simulink model "sys"  (R2024a)
settings: Solver=VariableStepAuto  StartTime=0.0  StopTime=2e-3  RelTol=1e-3
libraries: dspsigops x11, commdigbbndpm3 x1, commrandsrc3 x1, simulink x1
(part 1 of 2)
settings Model: Creator=abc  LastModifiedBy=abc

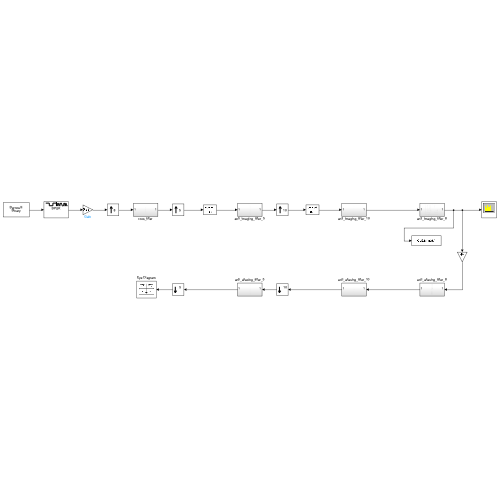
[thumbnail: Simulink's stored preview of the top-level diagram]
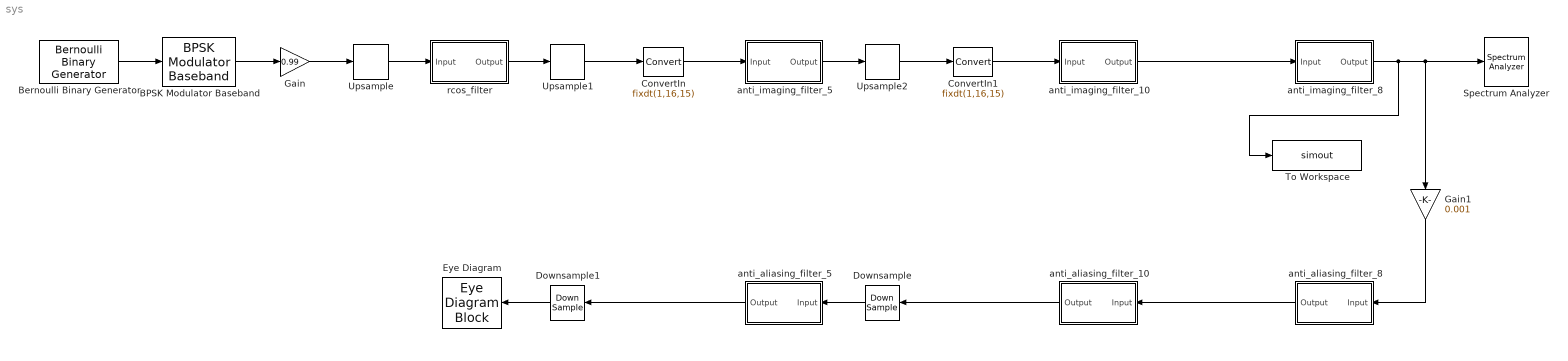
== system sys ==
  BPSK Modulator Baseband : commdigbbndpm3/BPSK Modulator Baseband  Ph=0  outDtype=double  outWordLen=16  outUDDataType=sfix(16)  outFracLenMode=Best precision  outFracLen=15  outDataTypeStr=double  outLastDataTypeStr=double
  Bernoulli Binary Generator : commrandsrc3/Bernoulli Binary Generator  ProbabilityOfZero=0.5  SeedSource=Auto  Seed=0  SampleTime=1/(450e3)  SamplesPerFrame=1  OutputDataType=double  SimulateUsing=Interpreted execution
  ConvertIn : DataTypeConversion  OutDataTypeStr=fixdt(1,16,15)  ConvertRealWorld=Stored Integer (SI)  RndMeth=Nearest
  ConvertIn1 : DataTypeConversion  OutDataTypeStr=fixdt(1,16,15)  ConvertRealWorld=Stored Integer (SI)  RndMeth=Nearest
  Downsample : DownSample  N=10  RateOptions=Allow multirate processing  AllowArbitraryFixedInput=on
  Downsample1 : DownSample  N=5  RateOptions=Allow multirate processing  AllowArbitraryFixedInput=on
  Eye Diagram : EyeDiagramBlock  WindowPosition=[302.000000,120.000000,800.000000,500.000000,]  ScopeFrameLocation=window  YLimits=[-2.8631442273035645,3.1513396510854363]  PlotImaginaryAxes=off
  Gain : Gain  Gain=0.99
  Gain1 : Gain  Gain=0.001
  Spectrum Analyzer : SpectrumAnalyzer  WindowPosition=[48.000000,117.000000,800.000000,500.000000,]  ScopeFrameLocation=window  SampleRateSource=Property  SampleRate=1  Span=3600000.0000000005  StartFrequency=-1800000.0000000002  StopFrequency=1800000.0000000002  YLimits=[-122.72965629,37.88911859]  ExpandToolstrip=on
  To Workspace : ToWorkspace  VariableName=simout  SampleTime=-1
      settings: Save2DSignal=2-D array (concatenate along first dimension)
  Upsample : dspsigops/Upsample  FactorSource=Dialog parameter  N=8  Nmax=16  phase=0  InputProcessing=Columns as channels (frame based)  RateOptions=Allow multirate processing  ic=0  mode=Unused parameter value
  Upsample1 : dspsigops/Upsample  FactorSource=Dialog parameter  N=5  Nmax=16  phase=0  InputProcessing=Columns as channels (frame based)  RateOptions=Allow multirate processing  ic=0  mode=Unused parameter value
  Upsample2 : dspsigops/Upsample  FactorSource=Dialog parameter  N=10  Nmax=16  phase=0  InputProcessing=Columns as channels (frame based)  RateOptions=Allow multirate processing  ic=0  mode=Unused parameter value
  anti_aliasing_filter_10 : Subsystem  Tag=FilterWizardSubSystem
      settings: ErrorFcn=dspFilterRealizedInBasicElemsAlgLoopErrFcnCallback
  anti_aliasing_filter_5 : Subsystem  Tag=FilterWizardSubSystem
      settings: ErrorFcn=dspFilterRealizedInBasicElemsAlgLoopErrFcnCallback
  anti_aliasing_filter_8 : Subsystem  Tag=FilterWizardSubSystem
      settings: ErrorFcn=dspFilterRealizedInBasicElemsAlgLoopErrFcnCallback
  anti_imaging_filter_10 : Subsystem  Tag=FilterWizardSubSystem
      settings: ErrorFcn=dspFilterRealizedInBasicElemsAlgLoopErrFcnCallback
  anti_imaging_filter_5 : Subsystem  Tag=FilterWizardSubSystem
      settings: ErrorFcn=dspFilterRealizedInBasicElemsAlgLoopErrFcnCallback
  anti_imaging_filter_8 : Subsystem  Tag=FilterWizardSubSystem
      settings: ErrorFcn=dspFilterRealizedInBasicElemsAlgLoopErrFcnCallback
  rcos_filter : Subsystem  Tag=FilterWizardSubSystem
      settings: ErrorFcn=dspFilterRealizedInBasicElemsAlgLoopErrFcnCallback
  wires:
  Bernoulli Binary Generator/1 -> BPSK Modulator Baseband/1
  BPSK Modulator Baseband/1 -> Gain/1
  Upsample/1 -> rcos_filter/1(Input)
  rcos_filter/1(Output) -> Upsample1/1
  anti_imaging_filter_5/1(Output) -> Upsample2/1
  Downsample/1 -> anti_aliasing_filter_5/1(Input)
  anti_aliasing_filter_5/1(Output) -> Downsample1/1
  anti_aliasing_filter_8/1(Output) -> anti_aliasing_filter_10/1(Input)
  anti_aliasing_filter_10/1(Output) -> Downsample/1
  Gain/1 -> Upsample/1
  Upsample1/1 -> ConvertIn/1
  Upsample2/1 -> ConvertIn1/1
  anti_imaging_filter_8/1(Output) -> To Workspace/1, Gain1/1, Spectrum Analyzer/1
  ConvertIn/1 -> anti_imaging_filter_5/1(Input)
  ConvertIn1/1 -> anti_imaging_filter_10/1(Input)
  Downsample1/1 -> Eye Diagram/1
  anti_imaging_filter_10/1(Output) -> anti_imaging_filter_8/1(Input)
  Gain1/1 -> anti_aliasing_filter_8/1(Input)

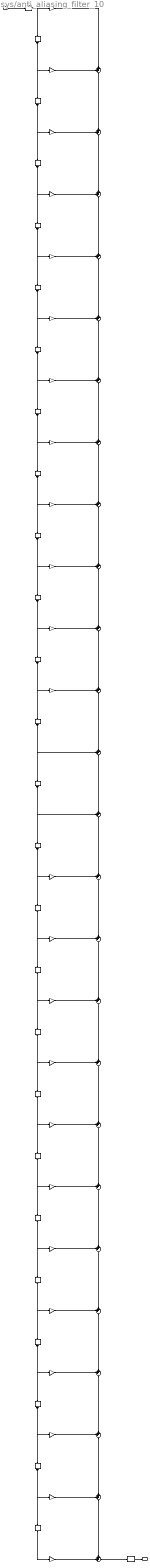
== system sys/anti_aliasing_filter_10 ==
  Input : Inport
  BodyDelay{2..26} (25 alike) : Delay  DelayLength=1  InitialCondition=0
  BodyLSum{2..26} (25 alike) : Sum  Inputs=++|  OutDataTypeStr=fixdt(1,35,30)  AccumDataTypeStr=fixdt(1,35,30)  RndMeth=Convergent
  ConvertIn : DataTypeConversion  OutDataTypeStr=fixdt(1,16,15)  RndMeth=Nearest
  ConvertOut : DataTypeConversion  OutDataTypeStr=fixdt(1,15,14)  RndMeth=Convergent  SaturateOnIntegerOverflow=off
  b(1) : Gain  Gain=0.0156626064233622506  ParamDataTypeStr=fixdt(1,16,15)  OutDataTypeStr=fixdt(1,31,30)  RndMeth=Convergent
  b(10) : Gain  Gain=0.784930628612014125  ParamDataTypeStr=fixdt(1,16,15)  OutDataTypeStr=fixdt(1,31,30)  RndMeth=Convergent
  b(11) : Gain  Gain=0.886772527356170293  ParamDataTypeStr=fixdt(1,16,15)  OutDataTypeStr=fixdt(1,31,30)  RndMeth=Convergent
  b(12) : Gain  Gain=0.960925295623340392  ParamDataTypeStr=fixdt(1,16,15)  OutDataTypeStr=fixdt(1,31,30)  RndMeth=Convergent
  b(15) : Gain  Gain=0.960925295623340392  ParamDataTypeStr=fixdt(1,16,15)  OutDataTypeStr=fixdt(1,31,30)  RndMeth=Convergent
  b(16) : Gain  Gain=0.886772527356170293  ParamDataTypeStr=fixdt(1,16,15)  OutDataTypeStr=fixdt(1,31,30)  RndMeth=Convergent
  b(17) : Gain  Gain=0.784930628612014125  ParamDataTypeStr=fixdt(1,16,15)  OutDataTypeStr=fixdt(1,31,30)  RndMeth=Convergent
  b(18) : Gain  Gain=0.665103266921935554  ParamDataTypeStr=fixdt(1,16,15)  OutDataTypeStr=fixdt(1,31,30)  RndMeth=Convergent
  b(19) : Gain  Gain=0.537919174813016099  ParamDataTypeStr=fixdt(1,16,15)  OutDataTypeStr=fixdt(1,31,30)  RndMeth=Convergent
  b(2) : Gain  Gain=0.0362761924333834043  ParamDataTypeStr=fixdt(1,16,15)  OutDataTypeStr=fixdt(1,31,30)  RndMeth=Convergent
  b(20) : Gain  Gain=0.413536705569194474  ParamDataTypeStr=fixdt(1,16,15)  OutDataTypeStr=fixdt(1,31,30)  RndMeth=Convergent
  b(21) : Gain  Gain=0.30040563304203749  ParamDataTypeStr=fixdt(1,16,15)  OutDataTypeStr=fixdt(1,31,30)  RndMeth=Convergent
  b(22) : Gain  Gain=0.204429372845306323  ParamDataTypeStr=fixdt(1,16,15)  OutDataTypeStr=fixdt(1,31,30)  RndMeth=Convergent
  b(23) : Gain  Gain=0.128628263180761093  ParamDataTypeStr=fixdt(1,16,15)  OutDataTypeStr=fixdt(1,31,30)  RndMeth=Convergent
  b(24) : Gain  Gain=0.0732387285445653402  ParamDataTypeStr=fixdt(1,16,15)  OutDataTypeStr=fixdt(1,31,30)  RndMeth=Convergent
  b(25) : Gain  Gain=0.0362761924333834043  ParamDataTypeStr=fixdt(1,16,15)  OutDataTypeStr=fixdt(1,31,30)  RndMeth=Convergent
  b(26) : Gain  Gain=0.0156626064233622506  ParamDataTypeStr=fixdt(1,16,15)  OutDataTypeStr=fixdt(1,31,30)  RndMeth=Convergent
  b(3) : Gain  Gain=0.0732387285445653402  ParamDataTypeStr=fixdt(1,16,15)  OutDataTypeStr=fixdt(1,31,30)  RndMeth=Convergent
  b(4) : Gain  Gain=0.128628263180761093  ParamDataTypeStr=fixdt(1,16,15)  OutDataTypeStr=fixdt(1,31,30)  RndMeth=Convergent
  b(5) : Gain  Gain=0.204429372845306323  ParamDataTypeStr=fixdt(1,16,15)  OutDataTypeStr=fixdt(1,31,30)  RndMeth=Convergent
  b(6) : Gain  Gain=0.30040563304203749  ParamDataTypeStr=fixdt(1,16,15)  OutDataTypeStr=fixdt(1,31,30)  RndMeth=Convergent
  b(7) : Gain  Gain=0.413536705569194474  ParamDataTypeStr=fixdt(1,16,15)  OutDataTypeStr=fixdt(1,31,30)  RndMeth=Convergent
  b(8) : Gain  Gain=0.537919174813016099  ParamDataTypeStr=fixdt(1,16,15)  OutDataTypeStr=fixdt(1,31,30)  RndMeth=Convergent
  b(9) : Gain  Gain=0.665103266921935554  ParamDataTypeStr=fixdt(1,16,15)  OutDataTypeStr=fixdt(1,31,30)  RndMeth=Convergent
  Output : Outport
  wires:
  Input/1 -> ConvertIn/1
  b(1)/1 -> BodyLSum2/2
  ConvertIn/1 -> b(1)/1, BodyDelay2/1
  BodyDelay2/1 -> b(2)/1, BodyDelay3/1
  b(2)/1 -> BodyLSum2/1
  BodyLSum2/1 -> BodyLSum3/2
  BodyDelay3/1 -> b(3)/1, BodyDelay4/1
  b(3)/1 -> BodyLSum3/1
  BodyLSum3/1 -> BodyLSum4/2
  BodyDelay4/1 -> b(4)/1, BodyDelay5/1
  b(4)/1 -> BodyLSum4/1
  BodyLSum4/1 -> BodyLSum5/2
  BodyDelay5/1 -> b(5)/1, BodyDelay6/1
  b(5)/1 -> BodyLSum5/1
  BodyLSum5/1 -> BodyLSum6/2
  BodyDelay6/1 -> b(6)/1, BodyDelay7/1
  b(6)/1 -> BodyLSum6/1
  BodyLSum6/1 -> BodyLSum7/2
  BodyDelay7/1 -> b(7)/1, BodyDelay8/1
  b(7)/1 -> BodyLSum7/1
  BodyLSum7/1 -> BodyLSum8/2
  BodyDelay8/1 -> b(8)/1, BodyDelay9/1
  b(8)/1 -> BodyLSum8/1
  BodyLSum8/1 -> BodyLSum9/2
  BodyDelay9/1 -> b(9)/1, BodyDelay10/1
  b(9)/1 -> BodyLSum9/1
  BodyLSum9/1 -> BodyLSum10/2
  BodyDelay10/1 -> b(10)/1, BodyDelay11/1
  b(10)/1 -> BodyLSum10/1
  BodyLSum10/1 -> BodyLSum11/2
  BodyDelay11/1 -> b(11)/1, BodyDelay12/1
  b(11)/1 -> BodyLSum11/1
  BodyLSum11/1 -> BodyLSum12/2
  BodyDelay12/1 -> b(12)/1, BodyDelay13/1
  b(12)/1 -> BodyLSum12/1
  BodyLSum12/1 -> BodyLSum13/2
  BodyDelay13/1 -> BodyLSum13/1, BodyDelay14/1
  BodyLSum13/1 -> BodyLSum14/2
  BodyDelay14/1 -> BodyLSum14/1, BodyDelay15/1
  BodyLSum14/1 -> BodyLSum15/2
  BodyDelay15/1 -> b(15)/1, BodyDelay16/1
  b(15)/1 -> BodyLSum15/1
  BodyLSum15/1 -> BodyLSum16/2
  BodyDelay16/1 -> b(16)/1, BodyDelay17/1
  b(16)/1 -> BodyLSum16/1
  BodyLSum16/1 -> BodyLSum17/2
  BodyDelay17/1 -> b(17)/1, BodyDelay18/1
  b(17)/1 -> BodyLSum17/1
  BodyLSum17/1 -> BodyLSum18/2
  BodyDelay18/1 -> b(18)/1, BodyDelay19/1
  b(18)/1 -> BodyLSum18/1
  BodyLSum18/1 -> BodyLSum19/2
  BodyDelay19/1 -> b(19)/1, BodyDelay20/1
  b(19)/1 -> BodyLSum19/1
  BodyLSum19/1 -> BodyLSum20/2
  BodyDelay20/1 -> b(20)/1, BodyDelay21/1
  b(20)/1 -> BodyLSum20/1
  BodyLSum20/1 -> BodyLSum21/2
  BodyDelay21/1 -> b(21)/1, BodyDelay22/1
  b(21)/1 -> BodyLSum21/1
  BodyLSum21/1 -> BodyLSum22/2
  BodyDelay22/1 -> b(22)/1, BodyDelay23/1
  b(22)/1 -> BodyLSum22/1
  BodyLSum22/1 -> BodyLSum23/2
  BodyDelay23/1 -> b(23)/1, BodyDelay24/1
  b(23)/1 -> BodyLSum23/1
  BodyLSum23/1 -> BodyLSum24/2
  BodyDelay24/1 -> b(24)/1, BodyDelay25/1
  b(24)/1 -> BodyLSum24/1
  BodyLSum24/1 -> BodyLSum25/2
  BodyDelay25/1 -> b(25)/1, BodyDelay26/1
  b(25)/1 -> BodyLSum25/1
  BodyLSum25/1 -> BodyLSum26/1
  BodyDelay26/1 -> b(26)/1
  b(26)/1 -> BodyLSum26/2
  BodyLSum26/1 -> ConvertOut/1
  ConvertOut/1 -> Output/1

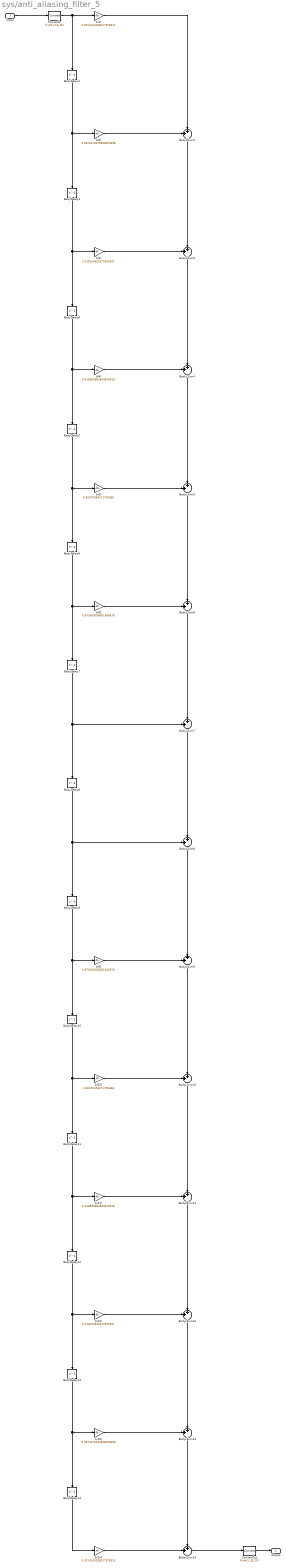
== system sys/anti_aliasing_filter_5 ==
  Input : Inport
  BodyDelay{2..14} (13 alike) : Delay  DelayLength=1  InitialCondition=0
  BodyLSum{2..14} (13 alike) : Sum  Inputs=++|  OutDataTypeStr=fixdt(1,33,29)  AccumDataTypeStr=fixdt(1,33,29)  RndMeth=Convergent
  ConvertIn : DataTypeConversion  OutDataTypeStr=fixdt(1,16,15)  RndMeth=Nearest
  ConvertOut : DataTypeConversion  OutDataTypeStr=fixdt(1,33,29)  RndMeth=Convergent  SaturateOnIntegerOverflow=off
  b(1) : Gain  Gain=0.0224233208217978312  ParamDataTypeStr=fixdt(1,16,14)  OutDataTypeStr=fixdt(1,31,29)  RndMeth=Convergent
  b(10) : Gain  Gain=0.65370494271794366  ParamDataTypeStr=fixdt(1,16,14)  OutDataTypeStr=fixdt(1,31,29)  RndMeth=Convergent
  b(11) : Gain  Gain=0.416892883843040518  ParamDataTypeStr=fixdt(1,16,14)  OutDataTypeStr=fixdt(1,31,29)  RndMeth=Convergent
  b(12) : Gain  Gain=0.218154593372955397  ParamDataTypeStr=fixdt(1,16,14)  OutDataTypeStr=fixdt(1,31,29)  RndMeth=Convergent
  b(13) : Gain  Gain=0.0873276240858359698  ParamDataTypeStr=fixdt(1,16,14)  OutDataTypeStr=fixdt(1,31,29)  RndMeth=Convergent
  b(14) : Gain  Gain=0.0224233208217978312  ParamDataTypeStr=fixdt(1,16,14)  OutDataTypeStr=fixdt(1,31,29)  RndMeth=Convergent
  b(2) : Gain  Gain=0.0873276240858359698  ParamDataTypeStr=fixdt(1,16,14)  OutDataTypeStr=fixdt(1,31,29)  RndMeth=Convergent
  b(3) : Gain  Gain=0.218154593372955397  ParamDataTypeStr=fixdt(1,16,14)  OutDataTypeStr=fixdt(1,31,29)  RndMeth=Convergent
  b(4) : Gain  Gain=0.416892883843040518  ParamDataTypeStr=fixdt(1,16,14)  OutDataTypeStr=fixdt(1,31,29)  RndMeth=Convergent
  b(5) : Gain  Gain=0.65370494271794366  ParamDataTypeStr=fixdt(1,16,14)  OutDataTypeStr=fixdt(1,31,29)  RndMeth=Convergent
  b(6) : Gain  Gain=0.870045056661949978  ParamDataTypeStr=fixdt(1,16,14)  OutDataTypeStr=fixdt(1,31,29)  RndMeth=Convergent
  b(9) : Gain  Gain=0.870045056661949978  ParamDataTypeStr=fixdt(1,16,14)  OutDataTypeStr=fixdt(1,31,29)  RndMeth=Convergent
  Output : Outport
  wires:
  Input/1 -> ConvertIn/1
  b(1)/1 -> BodyLSum2/2
  ConvertIn/1 -> b(1)/1, BodyDelay2/1
  BodyDelay2/1 -> b(2)/1, BodyDelay3/1
  b(2)/1 -> BodyLSum2/1
  BodyLSum2/1 -> BodyLSum3/2
  BodyDelay3/1 -> b(3)/1, BodyDelay4/1
  b(3)/1 -> BodyLSum3/1
  BodyLSum3/1 -> BodyLSum4/2
  BodyDelay4/1 -> b(4)/1, BodyDelay5/1
  b(4)/1 -> BodyLSum4/1
  BodyLSum4/1 -> BodyLSum5/2
  BodyDelay5/1 -> b(5)/1, BodyDelay6/1
  b(5)/1 -> BodyLSum5/1
  BodyLSum5/1 -> BodyLSum6/2
  BodyDelay6/1 -> b(6)/1, BodyDelay7/1
  b(6)/1 -> BodyLSum6/1
  BodyLSum6/1 -> BodyLSum7/2
  BodyDelay7/1 -> BodyLSum7/1, BodyDelay8/1
  BodyLSum7/1 -> BodyLSum8/2
  BodyDelay8/1 -> BodyLSum8/1, BodyDelay9/1
  BodyLSum8/1 -> BodyLSum9/2
  BodyDelay9/1 -> b(9)/1, BodyDelay10/1
  b(9)/1 -> BodyLSum9/1
  BodyLSum9/1 -> BodyLSum10/2
  BodyDelay10/1 -> b(10)/1, BodyDelay11/1
  b(10)/1 -> BodyLSum10/1
  BodyLSum10/1 -> BodyLSum11/2
  BodyDelay11/1 -> b(11)/1, BodyDelay12/1
  b(11)/1 -> BodyLSum11/1
  BodyLSum11/1 -> BodyLSum12/2
  BodyDelay12/1 -> b(12)/1, BodyDelay13/1
  b(12)/1 -> BodyLSum12/1
  BodyLSum12/1 -> BodyLSum13/2
  BodyDelay13/1 -> b(13)/1, BodyDelay14/1
  b(13)/1 -> BodyLSum13/1
  BodyLSum13/1 -> BodyLSum14/1
  BodyDelay14/1 -> b(14)/1
  b(14)/1 -> BodyLSum14/2
  BodyLSum14/1 -> ConvertOut/1
  ConvertOut/1 -> Output/1

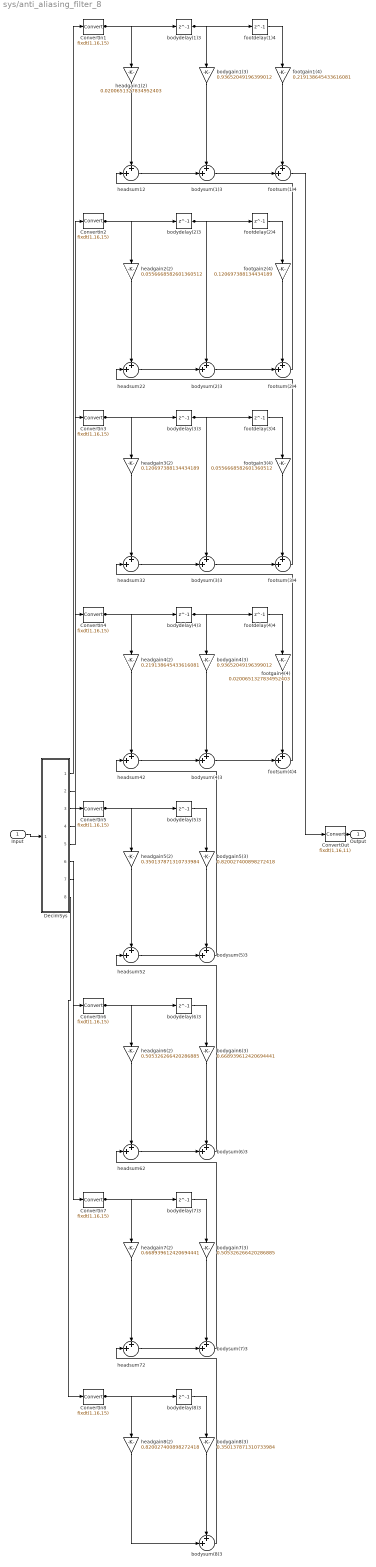
== system sys/anti_aliasing_filter_8 ==
  Input : Inport
  ConvertIn{1..8} (8 alike) : DataTypeConversion  OutDataTypeStr=fixdt(1,16,15)  RndMeth=Nearest
  ConvertOut : DataTypeConversion  OutDataTypeStr=fixdt(1,16,11)  RndMeth=Convergent  SaturateOnIntegerOverflow=off
  DecimSys : Subsystem  Tag=FilterWizardDecimatorCommutator
  bodydelay(1)3 : Delay  DelayLength=1  InitialCondition=0
  bodydelay(2)3 : Delay  DelayLength=1  InitialCondition=0
  bodydelay(3)3 : Delay  DelayLength=1  InitialCondition=0
  bodydelay(4)3 : Delay  DelayLength=1  InitialCondition=0
  bodydelay(5)3 : Delay  DelayLength=1  InitialCondition=0
  bodydelay(6)3 : Delay  DelayLength=1  InitialCondition=0
  bodydelay(7)3 : Delay  DelayLength=1  InitialCondition=0
  bodydelay(8)3 : Delay  DelayLength=1  InitialCondition=0
  bodygain1(3) : Gain  Gain=0.93652049196399012  ParamDataTypeStr=fixdt(1,16,15)  OutDataTypeStr=fixdt(1,31,30)  RndMeth=Convergent
  bodygain4(3) : Gain  Gain=0.93652049196399012  ParamDataTypeStr=fixdt(1,16,15)  OutDataTypeStr=fixdt(1,31,30)  RndMeth=Convergent
  bodygain5(3) : Gain  Gain=0.820027400898272418  ParamDataTypeStr=fixdt(1,16,15)  OutDataTypeStr=fixdt(1,31,30)  RndMeth=Convergent
  bodygain6(3) : Gain  Gain=0.668939612420694441  ParamDataTypeStr=fixdt(1,16,15)  OutDataTypeStr=fixdt(1,31,30)  RndMeth=Convergent
  bodygain7(3) : Gain  Gain=0.505326266420286885  ParamDataTypeStr=fixdt(1,16,15)  OutDataTypeStr=fixdt(1,31,30)  RndMeth=Convergent
  bodygain8(3) : Gain  Gain=0.350137871310733984  ParamDataTypeStr=fixdt(1,16,15)  OutDataTypeStr=fixdt(1,31,30)  RndMeth=Convergent
  bodysum(1)3 : Sum  Inputs=++|  OutDataTypeStr=fixdt(1,35,30)  AccumDataTypeStr=fixdt(1,35,30)  RndMeth=Convergent
  bodysum(2)3 : Sum  Inputs=++|  OutDataTypeStr=fixdt(1,35,30)  AccumDataTypeStr=fixdt(1,35,30)  RndMeth=Convergent
  bodysum(3)3 : Sum  Inputs=++|  OutDataTypeStr=fixdt(1,35,30)  AccumDataTypeStr=fixdt(1,35,30)  RndMeth=Convergent
  bodysum(4)3 : Sum  Inputs=++|  OutDataTypeStr=fixdt(1,35,30)  AccumDataTypeStr=fixdt(1,35,30)  RndMeth=Convergent
  bodysum(5)3 : Sum  Inputs=++|  OutDataTypeStr=fixdt(1,35,30)  AccumDataTypeStr=fixdt(1,35,30)  RndMeth=Convergent
  bodysum(6)3 : Sum  Inputs=++|  OutDataTypeStr=fixdt(1,35,30)  AccumDataTypeStr=fixdt(1,35,30)  RndMeth=Convergent
  bodysum(7)3 : Sum  Inputs=++|  OutDataTypeStr=fixdt(1,35,30)  AccumDataTypeStr=fixdt(1,35,30)  RndMeth=Convergent
  bodysum(8)3 : Sum  Inputs=++|  OutDataTypeStr=fixdt(1,35,30)  AccumDataTypeStr=fixdt(1,35,30)  RndMeth=Convergent
  footdelay(1)4 : Delay  DelayLength=1  InitialCondition=0
  footdelay(2)4 : Delay  DelayLength=1  InitialCondition=0
  footdelay(3)4 : Delay  DelayLength=1  InitialCondition=0
  footdelay(4)4 : Delay  DelayLength=1  InitialCondition=0
  footgain1(4) : Gain  Gain=0.219138645433616081  ParamDataTypeStr=fixdt(1,16,15)  OutDataTypeStr=fixdt(1,31,30)  RndMeth=Convergent
  footgain2(4) : Gain  Gain=0.120697388134434189  ParamDataTypeStr=fixdt(1,16,15)  OutDataTypeStr=fixdt(1,31,30)  RndMeth=Convergent
  footgain3(4) : Gain  Gain=0.0556668582601360512  ParamDataTypeStr=fixdt(1,16,15)  OutDataTypeStr=fixdt(1,31,30)  RndMeth=Convergent
  footgain4(4) : Gain  Gain=0.0200651327834952403  ParamDataTypeStr=fixdt(1,16,15)  OutDataTypeStr=fixdt(1,31,30)  RndMeth=Convergent
  footsum(1)4 : Sum  Inputs=++|  OutDataTypeStr=fixdt(1,35,30)  AccumDataTypeStr=fixdt(1,35,30)  RndMeth=Convergent
  footsum(2)4 : Sum  Inputs=++|  OutDataTypeStr=fixdt(1,35,30)  AccumDataTypeStr=fixdt(1,35,30)  RndMeth=Convergent
  footsum(3)4 : Sum  Inputs=++|  OutDataTypeStr=fixdt(1,35,30)  AccumDataTypeStr=fixdt(1,35,30)  RndMeth=Convergent
  footsum(4)4 : Sum  Inputs=++|  OutDataTypeStr=fixdt(1,35,30)  AccumDataTypeStr=fixdt(1,35,30)  RndMeth=Convergent
  headgain1(2) : Gain  Gain=0.0200651327834952403  ParamDataTypeStr=fixdt(1,16,15)  OutDataTypeStr=fixdt(1,31,30)  RndMeth=Convergent
  headgain2(2) : Gain  Gain=0.0556668582601360512  ParamDataTypeStr=fixdt(1,16,15)  OutDataTypeStr=fixdt(1,31,30)  RndMeth=Convergent
  headgain3(2) : Gain  Gain=0.120697388134434189  ParamDataTypeStr=fixdt(1,16,15)  OutDataTypeStr=fixdt(1,31,30)  RndMeth=Convergent
  headgain4(2) : Gain  Gain=0.219138645433616081  ParamDataTypeStr=fixdt(1,16,15)  OutDataTypeStr=fixdt(1,31,30)  RndMeth=Convergent
  headgain5(2) : Gain  Gain=0.350137871310733984  ParamDataTypeStr=fixdt(1,16,15)  OutDataTypeStr=fixdt(1,31,30)  RndMeth=Convergent
  headgain6(2) : Gain  Gain=0.505326266420286885  ParamDataTypeStr=fixdt(1,16,15)  OutDataTypeStr=fixdt(1,31,30)  RndMeth=Convergent
  headgain7(2) : Gain  Gain=0.668939612420694441  ParamDataTypeStr=fixdt(1,16,15)  OutDataTypeStr=fixdt(1,31,30)  RndMeth=Convergent
  headgain8(2) : Gain  Gain=0.820027400898272418  ParamDataTypeStr=fixdt(1,16,15)  OutDataTypeStr=fixdt(1,31,30)  RndMeth=Convergent
  headsum{12,22,32,42,52,62,72} (7 alike) : Sum  Inputs=++|  OutDataTypeStr=fixdt(1,35,30)  AccumDataTypeStr=fixdt(1,35,30)  RndMeth=Convergent
  Output : Outport
  wires:
  Input/1 -> DecimSys/1(input)
  DecimSys/1(output1) -> ConvertIn1/1
  DecimSys/2(output2) -> ConvertIn2/1
  DecimSys/3(output3) -> ConvertIn3/1
  DecimSys/4(output4) -> ConvertIn4/1
  DecimSys/5(output5) -> ConvertIn5/1
  DecimSys/6(output6) -> ConvertIn6/1
  DecimSys/7(output7) -> ConvertIn7/1
  DecimSys/8(output8) -> ConvertIn8/1
  ConvertIn1/1 -> headgain1(2)/1, bodydelay(1)3/1
  ConvertIn2/1 -> headgain2(2)/1, bodydelay(2)3/1
  ConvertIn3/1 -> headgain3(2)/1, bodydelay(3)3/1
  ConvertIn4/1 -> headgain4(2)/1, bodydelay(4)3/1
  ConvertIn5/1 -> headgain5(2)/1, bodydelay(5)3/1
  ConvertIn6/1 -> headgain6(2)/1, bodydelay(6)3/1
  ConvertIn7/1 -> headgain7(2)/1, bodydelay(7)3/1
  ConvertIn8/1 -> headgain8(2)/1, bodydelay(8)3/1
  headgain1(2)/1 -> headsum12/1
  headgain2(2)/1 -> headsum22/1
  headgain3(2)/1 -> headsum32/1
  headgain4(2)/1 -> headsum42/1
  headgain5(2)/1 -> headsum52/1
  headgain6(2)/1 -> headsum62/1
  headgain7(2)/1 -> headsum72/1
  headgain8(2)/1 -> bodysum(8)3/2
  headsum12/1 -> bodysum(1)3/2
  headsum22/1 -> bodysum(2)3/2
  headsum32/1 -> bodysum(3)3/2
  headsum42/1 -> bodysum(4)3/2
  headsum52/1 -> bodysum(5)3/2
  headsum62/1 -> bodysum(6)3/2
  headsum72/1 -> bodysum(7)3/2
  bodygain1(3)/1 -> bodysum(1)3/1
  bodygain4(3)/1 -> bodysum(4)3/1
  bodygain5(3)/1 -> bodysum(5)3/1
  bodygain6(3)/1 -> bodysum(6)3/1
  bodygain7(3)/1 -> bodysum(7)3/1
  bodygain8(3)/1 -> bodysum(8)3/1
  bodysum(1)3/1 -> footsum(1)4/2
  bodysum(2)3/1 -> footsum(2)4/2
  bodysum(3)3/1 -> footsum(3)4/2
  bodysum(4)3/1 -> footsum(4)4/2
  bodysum(5)3/1 -> headsum42/2
  bodysum(6)3/1 -> headsum52/2
  bodysum(7)3/1 -> headsum62/2
  bodysum(8)3/1 -> headsum72/2
  bodydelay(1)3/1 -> bodygain1(3)/1, footdelay(1)4/1
  bodydelay(2)3/1 -> bodysum(2)3/1, footdelay(2)4/1
  bodydelay(3)3/1 -> bodysum(3)3/1, footdelay(3)4/1
  bodydelay(4)3/1 -> bodygain4(3)/1, footdelay(4)4/1
  bodydelay(5)3/1 -> bodygain5(3)/1
  bodydelay(6)3/1 -> bodygain6(3)/1
  bodydelay(7)3/1 -> bodygain7(3)/1
  bodydelay(8)3/1 -> bodygain8(3)/1
  footgain1(4)/1 -> footsum(1)4/1
  footgain2(4)/1 -> footsum(2)4/1
  footgain3(4)/1 -> footsum(3)4/1
  footgain4(4)/1 -> footsum(4)4/1
  footsum(1)4/1 -> ConvertOut/1
  footsum(2)4/1 -> headsum12/2
  footsum(3)4/1 -> headsum22/2
  footsum(4)4/1 -> headsum32/2
  footdelay(1)4/1 -> footgain1(4)/1
  footdelay(2)4/1 -> footgain2(4)/1
  footdelay(3)4/1 -> footgain3(4)/1
  footdelay(4)4/1 -> footgain4(4)/1
  ConvertOut/1 -> Output/1

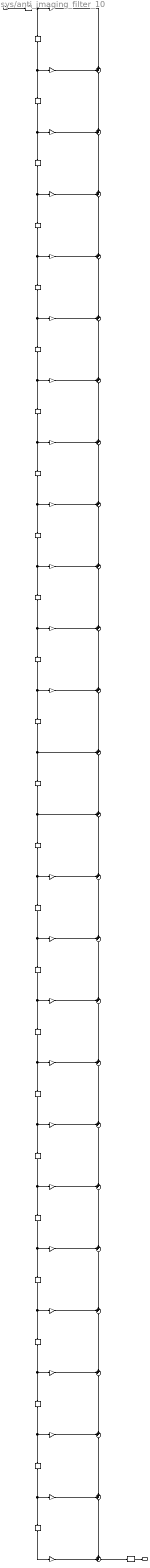
== system sys/anti_imaging_filter_10 ==
  Input : Inport
  BodyDelay{2..26} (25 alike) : Delay  DelayLength=1  InitialCondition=0  InputProcessing=Columns as channels (frame based)
  BodyLSum{2..26} (25 alike) : Sum  Inputs=++|  OutDataTypeStr=fixdt(1,35,30)  AccumDataTypeStr=fixdt(1,35,30)  RndMeth=Convergent
  ConvertIn : DataTypeConversion  OutDataTypeStr=fixdt(1,16,15)  RndMeth=Nearest
  ConvertOut : DataTypeConversion  OutDataTypeStr=fixdt(1,16,15)  RndMeth=Convergent  SaturateOnIntegerOverflow=off
  b(1) : Gain  Gain=0.0156626064233622506  ParamDataTypeStr=fixdt(1,16,15)  OutDataTypeStr=fixdt(1,31,30)  RndMeth=Convergent
  b(10) : Gain  Gain=0.784930628612014125  ParamDataTypeStr=fixdt(1,16,15)  OutDataTypeStr=fixdt(1,31,30)  RndMeth=Convergent
  b(11) : Gain  Gain=0.886772527356170293  ParamDataTypeStr=fixdt(1,16,15)  OutDataTypeStr=fixdt(1,31,30)  RndMeth=Convergent
  b(12) : Gain  Gain=0.960925295623340392  ParamDataTypeStr=fixdt(1,16,15)  OutDataTypeStr=fixdt(1,31,30)  RndMeth=Convergent
  b(15) : Gain  Gain=0.960925295623340392  ParamDataTypeStr=fixdt(1,16,15)  OutDataTypeStr=fixdt(1,31,30)  RndMeth=Convergent
  b(16) : Gain  Gain=0.886772527356170293  ParamDataTypeStr=fixdt(1,16,15)  OutDataTypeStr=fixdt(1,31,30)  RndMeth=Convergent
  b(17) : Gain  Gain=0.784930628612014125  ParamDataTypeStr=fixdt(1,16,15)  OutDataTypeStr=fixdt(1,31,30)  RndMeth=Convergent
  b(18) : Gain  Gain=0.665103266921935554  ParamDataTypeStr=fixdt(1,16,15)  OutDataTypeStr=fixdt(1,31,30)  RndMeth=Convergent
  b(19) : Gain  Gain=0.537919174813016099  ParamDataTypeStr=fixdt(1,16,15)  OutDataTypeStr=fixdt(1,31,30)  RndMeth=Convergent
  b(2) : Gain  Gain=0.0362761924333834043  ParamDataTypeStr=fixdt(1,16,15)  OutDataTypeStr=fixdt(1,31,30)  RndMeth=Convergent
  b(20) : Gain  Gain=0.413536705569194474  ParamDataTypeStr=fixdt(1,16,15)  OutDataTypeStr=fixdt(1,31,30)  RndMeth=Convergent
  b(21) : Gain  Gain=0.30040563304203749  ParamDataTypeStr=fixdt(1,16,15)  OutDataTypeStr=fixdt(1,31,30)  RndMeth=Convergent
  b(22) : Gain  Gain=0.204429372845306323  ParamDataTypeStr=fixdt(1,16,15)  OutDataTypeStr=fixdt(1,31,30)  RndMeth=Convergent
  b(23) : Gain  Gain=0.128628263180761093  ParamDataTypeStr=fixdt(1,16,15)  OutDataTypeStr=fixdt(1,31,30)  RndMeth=Convergent
  b(24) : Gain  Gain=0.0732387285445653402  ParamDataTypeStr=fixdt(1,16,15)  OutDataTypeStr=fixdt(1,31,30)  RndMeth=Convergent
  b(25) : Gain  Gain=0.0362761924333834043  ParamDataTypeStr=fixdt(1,16,15)  OutDataTypeStr=fixdt(1,31,30)  RndMeth=Convergent
  b(26) : Gain  Gain=0.0156626064233622506  ParamDataTypeStr=fixdt(1,16,15)  OutDataTypeStr=fixdt(1,31,30)  RndMeth=Convergent
  b(3) : Gain  Gain=0.0732387285445653402  ParamDataTypeStr=fixdt(1,16,15)  OutDataTypeStr=fixdt(1,31,30)  RndMeth=Convergent
  b(4) : Gain  Gain=0.128628263180761093  ParamDataTypeStr=fixdt(1,16,15)  OutDataTypeStr=fixdt(1,31,30)  RndMeth=Convergent
  b(5) : Gain  Gain=0.204429372845306323  ParamDataTypeStr=fixdt(1,16,15)  OutDataTypeStr=fixdt(1,31,30)  RndMeth=Convergent
  b(6) : Gain  Gain=0.30040563304203749  ParamDataTypeStr=fixdt(1,16,15)  OutDataTypeStr=fixdt(1,31,30)  RndMeth=Convergent
  b(7) : Gain  Gain=0.413536705569194474  ParamDataTypeStr=fixdt(1,16,15)  OutDataTypeStr=fixdt(1,31,30)  RndMeth=Convergent
  b(8) : Gain  Gain=0.537919174813016099  ParamDataTypeStr=fixdt(1,16,15)  OutDataTypeStr=fixdt(1,31,30)  RndMeth=Convergent
  b(9) : Gain  Gain=0.665103266921935554  ParamDataTypeStr=fixdt(1,16,15)  OutDataTypeStr=fixdt(1,31,30)  RndMeth=Convergent
  Output : Outport
  wires:
  Input/1 -> ConvertIn/1
  b(1)/1 -> BodyLSum2/2
  ConvertIn/1 -> b(1)/1, BodyDelay2/1
  BodyDelay2/1 -> b(2)/1, BodyDelay3/1
  b(2)/1 -> BodyLSum2/1
  BodyLSum2/1 -> BodyLSum3/2
  BodyDelay3/1 -> b(3)/1, BodyDelay4/1
  b(3)/1 -> BodyLSum3/1
  BodyLSum3/1 -> BodyLSum4/2
  BodyDelay4/1 -> b(4)/1, BodyDelay5/1
  b(4)/1 -> BodyLSum4/1
  BodyLSum4/1 -> BodyLSum5/2
  BodyDelay5/1 -> b(5)/1, BodyDelay6/1
  b(5)/1 -> BodyLSum5/1
  BodyLSum5/1 -> BodyLSum6/2
  BodyDelay6/1 -> b(6)/1, BodyDelay7/1
  b(6)/1 -> BodyLSum6/1
  BodyLSum6/1 -> BodyLSum7/2
  BodyDelay7/1 -> b(7)/1, BodyDelay8/1
  b(7)/1 -> BodyLSum7/1
  BodyLSum7/1 -> BodyLSum8/2
  BodyDelay8/1 -> b(8)/1, BodyDelay9/1
  b(8)/1 -> BodyLSum8/1
  BodyLSum8/1 -> BodyLSum9/2
  BodyDelay9/1 -> b(9)/1, BodyDelay10/1
  b(9)/1 -> BodyLSum9/1
  BodyLSum9/1 -> BodyLSum10/2
  BodyDelay10/1 -> b(10)/1, BodyDelay11/1
  b(10)/1 -> BodyLSum10/1
  BodyLSum10/1 -> BodyLSum11/2
  BodyDelay11/1 -> b(11)/1, BodyDelay12/1
  b(11)/1 -> BodyLSum11/1
  BodyLSum11/1 -> BodyLSum12/2
  BodyDelay12/1 -> b(12)/1, BodyDelay13/1
  b(12)/1 -> BodyLSum12/1
  BodyLSum12/1 -> BodyLSum13/2
  BodyDelay13/1 -> BodyLSum13/1, BodyDelay14/1
  BodyLSum13/1 -> BodyLSum14/2
  BodyDelay14/1 -> BodyLSum14/1, BodyDelay15/1
  BodyLSum14/1 -> BodyLSum15/2
  BodyDelay15/1 -> b(15)/1, BodyDelay16/1
  b(15)/1 -> BodyLSum15/1
  BodyLSum15/1 -> BodyLSum16/2
  BodyDelay16/1 -> b(16)/1, BodyDelay17/1
  b(16)/1 -> BodyLSum16/1
  BodyLSum16/1 -> BodyLSum17/2
  BodyDelay17/1 -> b(17)/1, BodyDelay18/1
  b(17)/1 -> BodyLSum17/1
  BodyLSum17/1 -> BodyLSum18/2
  BodyDelay18/1 -> b(18)/1, BodyDelay19/1
  b(18)/1 -> BodyLSum18/1
  BodyLSum18/1 -> BodyLSum19/2
  BodyDelay19/1 -> b(19)/1, BodyDelay20/1
  b(19)/1 -> BodyLSum19/1
  BodyLSum19/1 -> BodyLSum20/2
  BodyDelay20/1 -> b(20)/1, BodyDelay21/1
  b(20)/1 -> BodyLSum20/1
  BodyLSum20/1 -> BodyLSum21/2
  BodyDelay21/1 -> b(21)/1, BodyDelay22/1
  b(21)/1 -> BodyLSum21/1
  BodyLSum21/1 -> BodyLSum22/2
  BodyDelay22/1 -> b(22)/1, BodyDelay23/1
  b(22)/1 -> BodyLSum22/1
  BodyLSum22/1 -> BodyLSum23/2
  BodyDelay23/1 -> b(23)/1, BodyDelay24/1
  b(23)/1 -> BodyLSum23/1
  BodyLSum23/1 -> BodyLSum24/2
  BodyDelay24/1 -> b(24)/1, BodyDelay25/1
  b(24)/1 -> BodyLSum24/1
  BodyLSum24/1 -> BodyLSum25/2
  BodyDelay25/1 -> b(25)/1, BodyDelay26/1
  b(25)/1 -> BodyLSum25/1
  BodyLSum25/1 -> BodyLSum26/1
  BodyDelay26/1 -> b(26)/1
  b(26)/1 -> BodyLSum26/2
  BodyLSum26/1 -> ConvertOut/1
  ConvertOut/1 -> Output/1

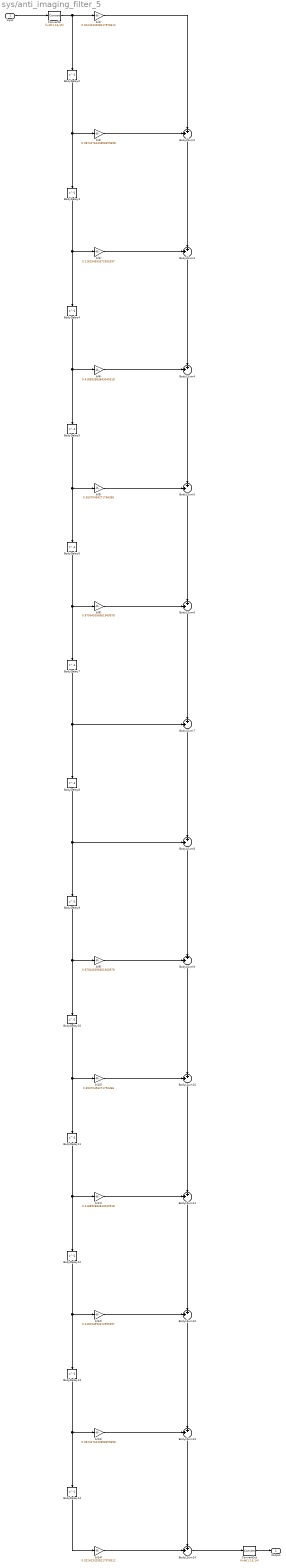
== system sys/anti_imaging_filter_5 ==
  Input : Inport
  BodyDelay{2..14} (13 alike) : Delay  DelayLength=1  InitialCondition=0  InputProcessing=Columns as channels (frame based)
  BodyLSum{2..14} (13 alike) : Sum  Inputs=++|  OutDataTypeStr=fixdt(1,34,30)  AccumDataTypeStr=fixdt(1,34,30)  RndMeth=Convergent
  ConvertIn : DataTypeConversion  OutDataTypeStr=fixdt(1,16,15)  ConvertRealWorld=Stored Integer (SI)  RndMeth=Nearest
  ConvertOut : DataTypeConversion  OutDataTypeStr=fixdt(1,16,14)  RndMeth=Convergent  SaturateOnIntegerOverflow=off
  b(1) : Gain  Gain=0.0224233208217978312  ParamDataTypeStr=fixdt(1,16,15)  OutDataTypeStr=fixdt(1,31,30)  RndMeth=Convergent
  b(10) : Gain  Gain=0.65370494271794366  ParamDataTypeStr=fixdt(1,16,15)  OutDataTypeStr=fixdt(1,31,30)  RndMeth=Convergent
  b(11) : Gain  Gain=0.416892883843040518  ParamDataTypeStr=fixdt(1,16,15)  OutDataTypeStr=fixdt(1,31,30)  RndMeth=Convergent
  b(12) : Gain  Gain=0.218154593372955397  ParamDataTypeStr=fixdt(1,16,15)  OutDataTypeStr=fixdt(1,31,30)  RndMeth=Convergent
  b(13) : Gain  Gain=0.0873276240858359698  ParamDataTypeStr=fixdt(1,16,15)  OutDataTypeStr=fixdt(1,31,30)  RndMeth=Convergent
  b(14) : Gain  Gain=0.0224233208217978312  ParamDataTypeStr=fixdt(1,16,15)  OutDataTypeStr=fixdt(1,31,30)  RndMeth=Convergent
  b(2) : Gain  Gain=0.0873276240858359698  ParamDataTypeStr=fixdt(1,16,15)  OutDataTypeStr=fixdt(1,31,30)  RndMeth=Convergent
  b(3) : Gain  Gain=0.218154593372955397  ParamDataTypeStr=fixdt(1,16,15)  OutDataTypeStr=fixdt(1,31,30)  RndMeth=Convergent
  b(4) : Gain  Gain=0.416892883843040518  ParamDataTypeStr=fixdt(1,16,15)  OutDataTypeStr=fixdt(1,31,30)  RndMeth=Convergent
  b(5) : Gain  Gain=0.65370494271794366  ParamDataTypeStr=fixdt(1,16,15)  OutDataTypeStr=fixdt(1,31,30)  RndMeth=Convergent
  b(6) : Gain  Gain=0.870045056661949978  ParamDataTypeStr=fixdt(1,16,15)  OutDataTypeStr=fixdt(1,31,30)  RndMeth=Convergent
  b(9) : Gain  Gain=0.870045056661949978  ParamDataTypeStr=fixdt(1,16,15)  OutDataTypeStr=fixdt(1,31,30)  RndMeth=Convergent
  Output : Outport
  wires:
  Input/1 -> ConvertIn/1
  b(1)/1 -> BodyLSum2/2
  ConvertIn/1 -> b(1)/1, BodyDelay2/1
  BodyDelay2/1 -> b(2)/1, BodyDelay3/1
  b(2)/1 -> BodyLSum2/1
  BodyLSum2/1 -> BodyLSum3/2
  BodyDelay3/1 -> b(3)/1, BodyDelay4/1
  b(3)/1 -> BodyLSum3/1
  BodyLSum3/1 -> BodyLSum4/2
  BodyDelay4/1 -> b(4)/1, BodyDelay5/1
  b(4)/1 -> BodyLSum4/1
  BodyLSum4/1 -> BodyLSum5/2
  BodyDelay5/1 -> b(5)/1, BodyDelay6/1
  b(5)/1 -> BodyLSum5/1
  BodyLSum5/1 -> BodyLSum6/2
  BodyDelay6/1 -> b(6)/1, BodyDelay7/1
  b(6)/1 -> BodyLSum6/1
  BodyLSum6/1 -> BodyLSum7/2
  BodyDelay7/1 -> BodyLSum7/1, BodyDelay8/1
  BodyLSum7/1 -> BodyLSum8/2
  BodyDelay8/1 -> BodyLSum8/1, BodyDelay9/1
  BodyLSum8/1 -> BodyLSum9/2
  BodyDelay9/1 -> b(9)/1, BodyDelay10/1
  b(9)/1 -> BodyLSum9/1
  BodyLSum9/1 -> BodyLSum10/2
  BodyDelay10/1 -> b(10)/1, BodyDelay11/1
  b(10)/1 -> BodyLSum10/1
  BodyLSum10/1 -> BodyLSum11/2
  BodyDelay11/1 -> b(11)/1, BodyDelay12/1
  b(11)/1 -> BodyLSum11/1
  BodyLSum11/1 -> BodyLSum12/2
  BodyDelay12/1 -> b(12)/1, BodyDelay13/1
  b(12)/1 -> BodyLSum12/1
  BodyLSum12/1 -> BodyLSum13/2
  BodyDelay13/1 -> b(13)/1, BodyDelay14/1
  b(13)/1 -> BodyLSum13/1
  BodyLSum13/1 -> BodyLSum14/1
  BodyDelay14/1 -> b(14)/1
  b(14)/1 -> BodyLSum14/2
  BodyLSum14/1 -> ConvertOut/1
  ConvertOut/1 -> Output/1

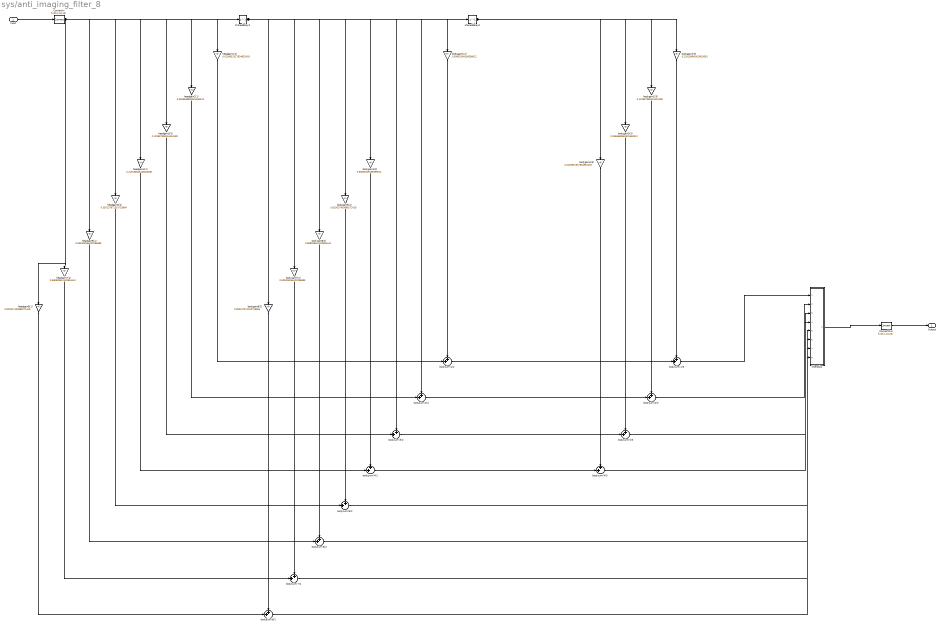
== system sys/anti_imaging_filter_8 ==
  Input : Inport
  ConvertIn : DataTypeConversion  OutDataTypeStr=fixdt(1,16,15)  RndMeth=Nearest
  ConvertOut : DataTypeConversion  OutDataTypeStr=fixdt(1,16,15)  RndMeth=Convergent  SaturateOnIntegerOverflow=off
  InterpSys : Subsystem  Tag=FilterWizardInterpolatorCommutator
  bodygain1(2) : Gain  Gain=0.93652049196399012  ParamDataTypeStr=fixdt(1,16,15)  OutDataTypeStr=fixdt(1,31,30)  RndMeth=Convergent
  bodygain1(3) : Gain  Gain=0.219138645433616081  ParamDataTypeStr=fixdt(1,16,15)  OutDataTypeStr=fixdt(1,31,30)  RndMeth=Convergent
  bodygain2(3) : Gain  Gain=0.120697388134434189  ParamDataTypeStr=fixdt(1,16,15)  OutDataTypeStr=fixdt(1,31,30)  RndMeth=Convergent
  bodygain3(3) : Gain  Gain=0.0556668582601360512  ParamDataTypeStr=fixdt(1,16,15)  OutDataTypeStr=fixdt(1,31,30)  RndMeth=Convergent
  bodygain4(2) : Gain  Gain=0.93652049196399012  ParamDataTypeStr=fixdt(1,16,15)  OutDataTypeStr=fixdt(1,31,30)  RndMeth=Convergent
  bodygain4(3) : Gain  Gain=0.0200651327834952403  ParamDataTypeStr=fixdt(1,16,15)  OutDataTypeStr=fixdt(1,31,30)  RndMeth=Convergent
  bodygain5(2) : Gain  Gain=0.820027400898272418  ParamDataTypeStr=fixdt(1,16,15)  OutDataTypeStr=fixdt(1,31,30)  RndMeth=Convergent
  bodygain6(2) : Gain  Gain=0.668939612420694441  ParamDataTypeStr=fixdt(1,16,15)  OutDataTypeStr=fixdt(1,31,30)  RndMeth=Convergent
  bodygain7(2) : Gain  Gain=0.505326266420286885  ParamDataTypeStr=fixdt(1,16,15)  OutDataTypeStr=fixdt(1,31,30)  RndMeth=Convergent
  bodygain8(2) : Gain  Gain=0.350137871310733984  ParamDataTypeStr=fixdt(1,16,15)  OutDataTypeStr=fixdt(1,31,30)  RndMeth=Convergent
  bodysum(1)2 : Sum  Inputs=++|  OutDataTypeStr=fixdt(1,35,30)  AccumDataTypeStr=fixdt(1,32,30)  RndMeth=Convergent
  bodysum(1)3 : Sum  Inputs=++|  OutDataTypeStr=fixdt(1,35,30)  AccumDataTypeStr=fixdt(1,32,30)  RndMeth=Convergent
  bodysum(2)2 : Sum  Inputs=++|  OutDataTypeStr=fixdt(1,35,30)  AccumDataTypeStr=fixdt(1,32,30)  RndMeth=Convergent
  bodysum(2)3 : Sum  Inputs=++|  OutDataTypeStr=fixdt(1,35,30)  AccumDataTypeStr=fixdt(1,32,30)  RndMeth=Convergent
  bodysum(3)2 : Sum  Inputs=++|  OutDataTypeStr=fixdt(1,35,30)  AccumDataTypeStr=fixdt(1,32,30)  RndMeth=Convergent
  bodysum(3)3 : Sum  Inputs=++|  OutDataTypeStr=fixdt(1,35,30)  AccumDataTypeStr=fixdt(1,32,30)  RndMeth=Convergent
  bodysum(4)2 : Sum  Inputs=++|  OutDataTypeStr=fixdt(1,35,30)  AccumDataTypeStr=fixdt(1,32,30)  RndMeth=Convergent
  bodysum(4)3 : Sum  Inputs=++|  OutDataTypeStr=fixdt(1,35,30)  AccumDataTypeStr=fixdt(1,32,30)  RndMeth=Convergent
  bodysum(5)2 : Sum  Inputs=++|  OutDataTypeStr=fixdt(1,35,30)  AccumDataTypeStr=fixdt(1,32,30)  RndMeth=Convergent
  bodysum(6)2 : Sum  Inputs=++|  OutDataTypeStr=fixdt(1,35,30)  AccumDataTypeStr=fixdt(1,32,30)  RndMeth=Convergent
  bodysum(7)2 : Sum  Inputs=++|  OutDataTypeStr=fixdt(1,35,30)  AccumDataTypeStr=fixdt(1,32,30)  RndMeth=Convergent
  bodysum(8)2 : Sum  Inputs=++|  OutDataTypeStr=fixdt(1,35,30)  AccumDataTypeStr=fixdt(1,32,30)  RndMeth=Convergent
  headgain1(1) : Gain  Gain=0.0200651327834952403  ParamDataTypeStr=fixdt(1,16,15)  OutDataTypeStr=fixdt(1,31,30)  RndMeth=Convergent
  headgain2(1) : Gain  Gain=0.0556668582601360512  ParamDataTypeStr=fixdt(1,16,15)  OutDataTypeStr=fixdt(1,31,30)  RndMeth=Convergent
  headgain3(1) : Gain  Gain=0.120697388134434189  ParamDataTypeStr=fixdt(1,16,15)  OutDataTypeStr=fixdt(1,31,30)  RndMeth=Convergent
  headgain4(1) : Gain  Gain=0.219138645433616081  ParamDataTypeStr=fixdt(1,16,15)  OutDataTypeStr=fixdt(1,31,30)  RndMeth=Convergent
  headgain5(1) : Gain  Gain=0.350137871310733984  ParamDataTypeStr=fixdt(1,16,15)  OutDataTypeStr=fixdt(1,31,30)  RndMeth=Convergent
  headgain6(1) : Gain  Gain=0.505326266420286885  ParamDataTypeStr=fixdt(1,16,15)  OutDataTypeStr=fixdt(1,31,30)  RndMeth=Convergent
  headgain7(1) : Gain  Gain=0.668939612420694441  ParamDataTypeStr=fixdt(1,16,15)  OutDataTypeStr=fixdt(1,31,30)  RndMeth=Convergent
  headgain8(1) : Gain  Gain=0.820027400898272418  ParamDataTypeStr=fixdt(1,16,15)  OutDataTypeStr=fixdt(1,31,30)  RndMeth=Convergent
  shareddelay2 : Delay  DelayLength=1  InitialCondition=0
  shareddelay3 : Delay  DelayLength=1  InitialCondition=0
  Output : Outport
  wires:
  headgain1(1)/1 -> bodysum(1)2/2
  headgain2(1)/1 -> bodysum(2)2/2
  headgain3(1)/1 -> bodysum(3)2/2
  headgain4(1)/1 -> bodysum(4)2/2
  headgain5(1)/1 -> bodysum(5)2/2
  headgain6(1)/1 -> bodysum(6)2/2
  headgain7(1)/1 -> bodysum(7)2/2
  headgain8(1)/1 -> bodysum(8)2/2
  Input/1 -> ConvertIn/1
  ConvertIn/1 -> headgain1(1)/1, headgain2(1)/1, headgain3(1)/1, headgain4(1)/1, headgain5(1)/1, headgain6(1)/1, headgain7(1)/1, headgain8(1)/1, shareddelay2/1
  bodygain1(2)/1 -> bodysum(1)2/1
  bodygain4(2)/1 -> bodysum(4)2/1
  bodygain5(2)/1 -> bodysum(5)2/1
  bodygain6(2)/1 -> bodysum(6)2/1
  bodygain7(2)/1 -> bodysum(7)2/1
  bodygain8(2)/1 -> bodysum(8)2/1
  bodysum(1)2/1 -> bodysum(1)3/2
  bodysum(2)2/1 -> bodysum(2)3/2
  bodysum(3)2/1 -> bodysum(3)3/2
  bodysum(4)2/1 -> bodysum(4)3/2
  bodysum(5)2/1 -> InterpSys/5(input5)
  bodysum(6)2/1 -> InterpSys/6(input6)
  bodysum(7)2/1 -> InterpSys/7(input7)
  bodysum(8)2/1 -> InterpSys/8(input8)
  shareddelay2/1 -> bodygain1(2)/1, bodysum(2)2/1, bodysum(3)2/1, bodygain4(2)/1, bodygain5(2)/1, bodygain6(2)/1, bodygain7(2)/1, bodygain8(2)/1, shareddelay3/1
  bodygain1(3)/1 -> bodysum(1)3/1
  bodygain2(3)/1 -> bodysum(2)3/1
  bodygain3(3)/1 -> bodysum(3)3/1
  bodygain4(3)/1 -> bodysum(4)3/1
  bodysum(1)3/1 -> InterpSys/1(input1)
  bodysum(2)3/1 -> InterpSys/2(input2)
  bodysum(3)3/1 -> InterpSys/3(input3)
  bodysum(4)3/1 -> InterpSys/4(input4)
  shareddelay3/1 -> bodygain1(3)/1, bodygain2(3)/1, bodygain3(3)/1, bodygain4(3)/1
  InterpSys/1(output) -> ConvertOut/1
  ConvertOut/1 -> Output/1
